simulink model "BP2_3"  (R2024a)
settings: Solver=VariableStepAuto  StartTime=0.0  StopTime=1500  RelTol=1e-3
libraries: neural x2
settings Model: Creator=yiqi2022  LastModifiedBy=51335
settings DebuggingCC: UnconnectedInputMsg=warning  UnconnectedOutputMsg=warning  UnconnectedLineMsg=warning
settings ModelReferenceCC: EnableRefExpFcnMdlSchedulingChecks=on
settings RTWCC: GPUComputeCapability=3.5  DLArmComputeVersion=19.05

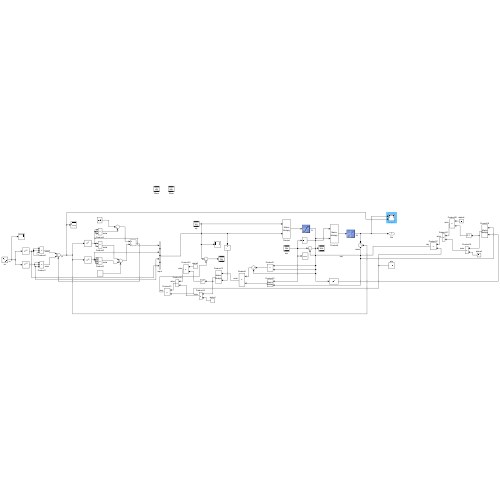
[thumbnail: Simulink's stored preview of the top-level diagram]
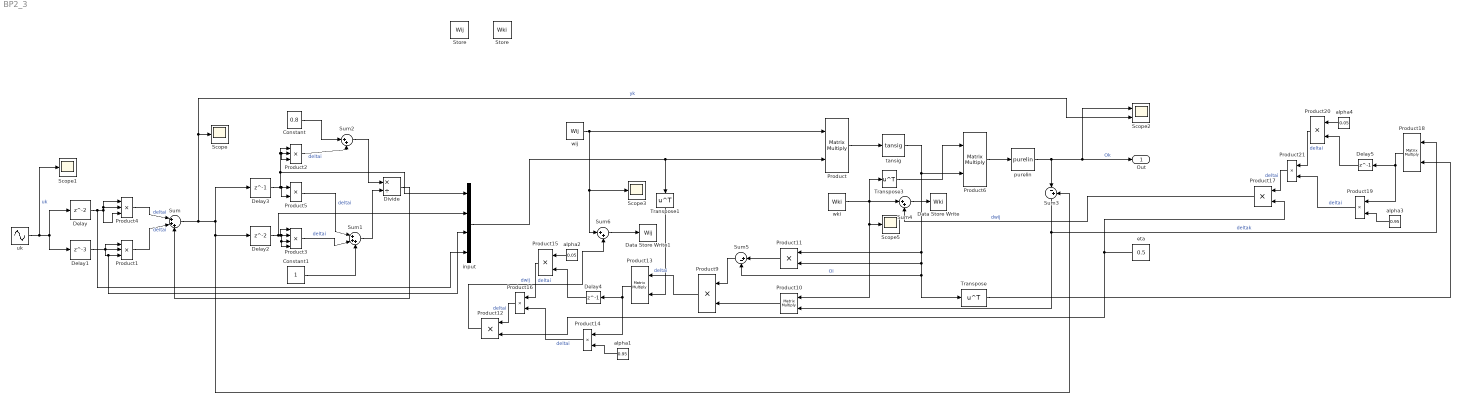
== system BP2_3 ==
  " Store " : DataStoreMemory  DataStoreName=Wki  ReadBeforeWriteMsg=warning  WriteAfterWriteMsg=warning  WriteAfterReadMsg=warning  InitialValue="[0.1832  -0.3349  0.7061  -0.1152  0.8087  -0.9336]"  ShowAdditionalParam=off
  Constant : Constant  Value=0.8
  Constant1 : Constant
  Data Store Write : DataStoreWrite  DataStoreName=Wki  IndexOptions=Index vector (dialog)  Indices=1  OutputSizes=1
  Data Store Write1 : DataStoreWrite  DataStoreName=Wij  IndexOptions=Index vector (dialog)  Indices=1  OutputSizes=1
  Delay : Delay
  Delay1 : Delay  DelayLength=3
  Delay2 : Delay
  Delay3 : Delay  DelayLength=1
  Delay4 : Delay  DelayLength=1
  Delay5 : Delay  DelayLength=1
  Divide : Product  Inputs=*/
  Product{,6,10,13,18} (5 alike) : Product  Multiplication=Matrix(*)
  Product1 : Product  Inputs=3
  Product{5,9,11..12,14..17,19..21} (11 alike) : Product
  Product2 : Product  Inputs=3
  Product3 : Product  Inputs=4
  Product4 : Product  Inputs=3
  Scope{,1,3,5} (4 alike) : Scope
  Scope2 : Scope  NumInputPorts=2
  "Store " : DataStoreMemory  DataStoreName=Wij  ReadBeforeWriteMsg=warning  WriteAfterWriteMsg=warning  WriteAfterReadMsg=warning  InitialValue="[ -0.8633    0.9231    0.1046    0.7128;   -0.1273    0.5248   -0.5638   -0.1951;   -0.6523   -0.9853    0.5447   -0.3640;   -0.9478    0.3601   -0.5439    0.2173;    0.9094    0.4119   -0.2583    0.8204;   -0.1388    0.2903    0.7819    0.8182]"  ShowAdditionalParam=off
  Sum : Sum  Inputs=|+++
  Sum1 : Sum  Inputs=|+++
  Sum2 : Sum  Inputs=|++
  Sum3 : Sum  Inputs=|-+
  Sum4 : Sum  Inputs=|++
  Sum5 : Sum  Inputs=|+-
  Sum6 : Sum  Inputs=|++
  Transpose : Math  Operator=transpose  SignedPower=on  RndMeth=Zero
  Transpose1 : Math  Operator=transpose  SignedPower=on  RndMeth=Zero
  Transpose3 : Math  Operator=transpose  SignedPower=on  RndMeth=Zero
  alpha1 : Constant  Value=0.95
  alpha2 : Constant  Value=0.05
  alpha3 : Constant  Value=0.95
  alpha4 : Constant  Value=0.05
  eta : Constant  Value=0.5
  input : Concatenate  NumInputs=4
  purelin : neural/Transfer Functions/purelin
  tansig : neural/Transfer Functions/tansig
  uk : Sin  Amplitude=0.8  Frequency=0.01  SampleTime=0
  wij : DataStoreRead  DataStoreName=Wij  SampleTime=0  IndexOptions=Index vector (dialog)  Indices=1  OutputSizes=1
  wki : DataStoreRead  DataStoreName=Wki  SampleTime=0  IndexOptions=Index vector (dialog)  Indices=1  OutputSizes=1
  Out : Outport  SampleTime=0
  wires:
  Sum2/1 -> Divide/1
  Product2/1 -> Sum2/2  "deltai"
  Product3/1 -> Sum1/2  "deltai"
  Constant/1 -> Sum2/1
  uk/1 -> Scope1/1, Delay/1, Delay1/1  "uk"
  Product4/1 -> Sum/1  "deltai"
  Product5/1 -> Sum1/1  "deltai"
  Delay1/1 -> input/3, Product1/3, Product1/2, Product1/1
  Product1/1 -> Sum/2  "deltai"
  Constant1/1 -> Sum1/3
  Divide/1 -> Sum/3
  Delay3/1 -> Product5/2, Product5/1, input/1, Product2/1, Product2/3, Product2/2
  Sum/1 -> Scope2/2, Scope/1, Sum3/2, Delay2/1, Delay3/1  "yk"
  Sum1/1 -> Divide/2
  Delay/1 -> input/4, Product4/2, Product4/1, Product4/3
  Product12/1 -> Sum6/2  "dwij"
  Transpose3/1 -> Product6/1
  Product9/1 -> Product13/1  "deltai"
  Product11/1 -> Sum5/1
  Sum5/1 -> Product9/1
  wki/1 -> Product10/1, Scope5/1, Transpose3/1, Sum4/1
  Sum3/1 -> Product18/1, Product10/2  "deltak"
  input/1 -> Product/2, Transpose1/1
  wij/1 -> Product/1, Scope3/1, Sum6/1
  eta/1 -> Product12/2, Product17/2
  Transpose/1 -> Product18/2
  Product/1 -> tansig/1
  Product10/1 -> Product9/2
  Sum4/1 -> Data Store Write/1
  Product6/1 -> purelin/1
  tansig/1 -> Sum5/2, Transpose/1, Product11/2, Product11/1, Product6/2  "Oi"
  Product13/1 -> Product14/1, Delay4/1
  purelin/1 -> Scope2/1, Out/1, Sum3/1  "Ok"
  Sum6/1 -> Data Store Write1/1
  Delay2/1 -> input/2, Product3/3, Product3/4, Product3/2, Product3/1
  Transpose1/1 -> Product13/2
  alpha1/1 -> Product14/2
  Delay4/1 -> Product15/2
  alpha2/1 -> Product15/1
  Product15/1 -> Product16/1  "deltai"
  Product14/1 -> Product16/2  "deltai"
  Product16/1 -> Product12/1  "deltai"
  Product21/1 -> Product17/1  "deltai"
  Delay5/1 -> Product20/2
  alpha3/1 -> Product19/2
  alpha4/1 -> Product20/1
  Product18/1 -> Product19/1, Delay5/1
  Product19/1 -> Product21/2  "deltai"
  Product20/1 -> Product21/1  "deltai"
  Product17/1 -> Sum4/2  "dwij"
